simulink model "testRead"  (Simulink 8.3)
settings: Solver=FixedStepDiscrete  StartTime=0.0  StopTime=inf  FixedStep=Ts  RelTol=1e-3
PreLoadFcn:
  | robotName = 'icub';
  | localName = 'SimulinkiCubGazeboSim';
  | Ts=0.01
  | ROBOT_DOF = 23;
InitFcn:
  | robotName = 'icub';
  | localName = 'read';
libraries: WBCLibrary x3
settings Model: Creator=iron  LastModifiedBy=daniele
settings OptimizationCC: ExpressionDepthLimit=2147483647
settings DebuggingCC: FcnCallInpInsideContextMsg=UseLocalSettings

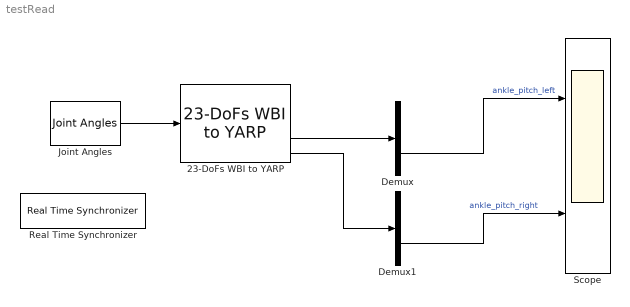
== system testRead ==
  23-DoFs WBI to YARP : WBCLibrary/Utilities/23-DoFs WBI to YARP
  Demux : Demux  Outputs=6
  Demux1 : Demux  Outputs=6
  Joint Angles : WBCLibrary/wholeBodyStates/Joint Angles  robotName=robotName  localName=localName
  Real Time Synchronizer : WBCLibrary/Utilities/Real Time Synchronizer  Priority=-10  threadPeriod=Ts
  Scope : Scope  NumInputPorts=2
      settings: ShowLegends=on  YMin=-7~-5  YMax=-0.5~-0.5
  wires:
  Joint Angles/1 -> 23-DoFs WBI to YARP/1
  23-DoFs WBI to YARP/4 -> Demux/1
  23-DoFs WBI to YARP/5 -> Demux1/1
  Demux/5 -> Scope/1  "ankle_pitch_left"
  Demux1/5 -> Scope/2  "ankle_pitch_right"
